simulink model "sldemo_bus_counter"  (Simulink 7.4)
settings: Solver=ode5  StartTime=0.0  StopTime=30  RelTol=1e-3
settings Model: Creator=The MathWorks Inc.  LastModifiedBy=alex  ExtModeAutoUpdateStatusClock=off
settings DataIOCC: SaveOutput=off  SaveTime=off  SignalLoggingName=logsOut
settings OptimizationCC: InlineParams=on  InlineInvariantSignals=on  InitFltsAndDblsToZero=on
settings DebuggingCC: SaveWithParameterizedLinksMsg=none  CheckExecutionContextPreStartOutputMsg=on  CheckExecutionContextRuntimeOutputMsg=on  SolverPrmCheckMsg=none  MultiTaskDSMMsg=warning  MultiTaskCondExecSysMsg=none  SigSpecEnsureSampleTimeMsg=none  StrictBusMsg=ErrorOnBusTreatedAsVector
settings HardwareCC: TargetHWDeviceType=32-bit Generic
settings ModelReferenceCC: UpdateModelReferenceTargets=IfOutOfDate
settings RTWCC: ProcessScript=grt_make_rtw_hook  IncludeERTFirstTime=on
settings CodeAppCC: MaxIdLength=100
settings GRTTargetCC: TargetFcnLib=ansi_tfl_tmw.mat

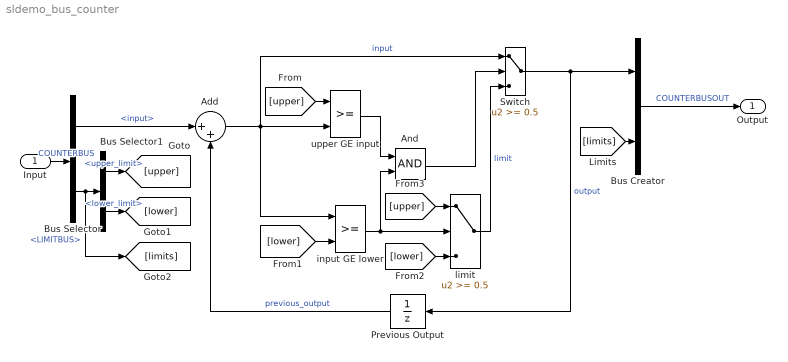
== system sldemo_bus_counter ==
  Input : Inport  UseBusObject=on  SampleTime=[0.10000000000000001,0]  OutDataType=sfix(16)  OutScaling=2^0
      settings: BusObject=COUNTERBUS
  " input GE lower" : RelationalOperator  Priority=1  InputSameDT=on
      settings: AttributesFormatString=\n
  " limit" : Switch  Threshold=0.5  SaturateOnIntegerOverflow=on  InputSameDT=on
  Add : Sum  Inputs=|++  OutDataType=sfix(16)  OutScaling=2^-10
  And : Logic
  Bus Creator : BusCreator  Inputs=2
  Bus Selector : BusSelector  OutputSignals=input,LIMITBUS
  Bus Selector1 : BusSelector  OutputSignals=upper_limit,lower_limit
  Previous Output : UnitDelay  SampleTime=-1
  Switch : Switch  Threshold=0.5  SaturateOnIntegerOverflow=on  InputSameDT=on
  upper GE input : RelationalOperator  Priority=0  InputSameDT=on
      settings: AttributesFormatString=\n
  Output : Outport  UseBusObject=on  SampleTime=[0.10000000000000001,0]  OutDataType=sfix(16)  OutScaling=2^0
      settings: BusObject=COUNTERBUSOUT
  wires:
  [limits] -> Bus Creator/2
  Bus Creator/1 -> Output/1  "COUNTERBUSOUT"
  Bus Selector1/2 -> [lower]  "<lower_limit>"
  Bus Selector1/1 -> [upper]  "<upper_limit>"
  Bus Selector/1 -> Add/1  "<input>"
  Bus Selector/2 -> Bus Selector1/1, [limits]  "<LIMITBUS>"
  Input/1 -> Bus Selector/1  "COUNTERBUS"
  Add/1 -> " input GE lower"/1, upper GE input/2, Switch/1  "input"
  And/1 -> Switch/2
  " input GE lower"/1 -> And/2, " limit"/2
  [lower] -> " input GE lower"/2
  [upper] -> upper GE input/1
  [lower] -> " limit"/3
  Previous Output/1 -> Add/2  "previous_output"
  upper GE input/1 -> And/1
  " limit"/1 -> Switch/3  "limit"
  Switch/1 -> Bus Creator/1, Previous Output/1  "output"
  [upper] -> " limit"/1
